simulink model "coord_test"  (R2013a)
settings: Solver=ode45  StartTime=0.0  StopTime=10.0  RelTol=1e-3
libraries: QuaternionLib x3
settings Model: Creator=EwingKang  LastModifiedBy=EwingKang

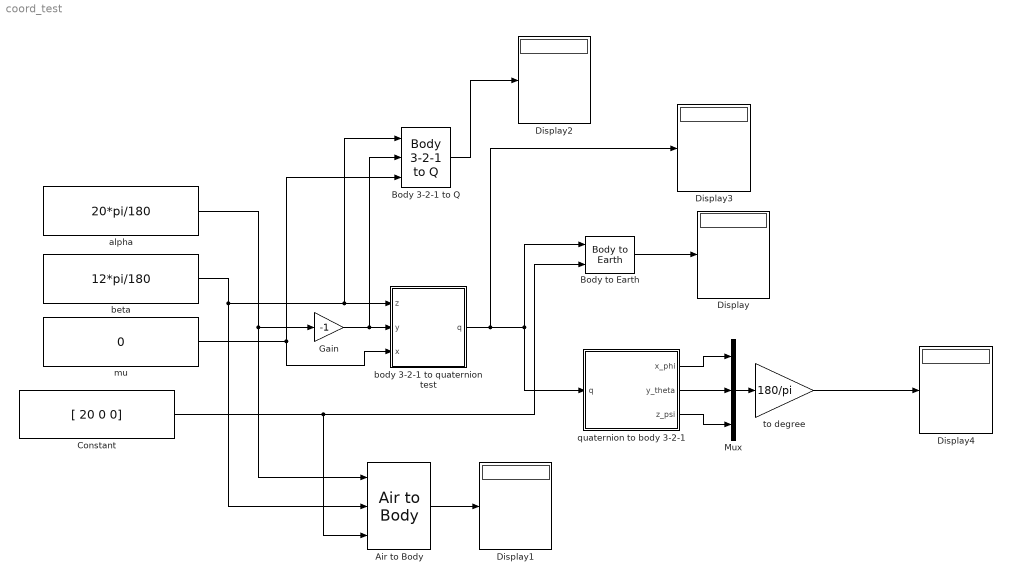
== system coord_test ==
  " quaternion to body 3-2-1" : MATLAB Function  TreatAsAtomicUnit=on
  Air to Body : QuaternionLib/Air to Body
  Body 3-2-1 to Q : QuaternionLib/Body 3-2-1 to Q
  Body to Earth : QuaternionLib/Body to Earth
  Constant : Constant  Value=[ 20 0 0]
  Display{,1..4} (5 alike) : Display
  Gain : Gain  Gain=-1
  Mux : Mux  Inputs=3
  alpha : Constant  Value=20*pi/180
  beta : Constant  Value=12*pi/180
  body 3-2-1 to quaternion test : MATLAB Function  TreatAsAtomicUnit=on
  mu : Constant  Value=0
  to degree : Gain  Gain=180/pi
  wires:
  body 3-2-1 to quaternion test/1(q) -> Display3/1, Body to Earth/1, " quaternion to body 3-2-1"/1(q)
  Constant/1 -> Air to Body/3, Body to Earth/2
  Body to Earth/1 -> Display/1
  Air to Body/1 -> Display1/1
  alpha/1 -> Air to Body/1, Gain/1
  beta/1 -> Body 3-2-1 to Q/1, body 3-2-1 to quaternion test/1(z), Air to Body/2
  mu/1 -> Body 3-2-1 to Q/3, body 3-2-1 to quaternion test/3(x)
  Gain/1 -> Body 3-2-1 to Q/2, body 3-2-1 to quaternion test/2(y)
  Body 3-2-1 to Q/1 -> Display2/1
  " quaternion to body 3-2-1"/2(y_theta) -> Mux/2
  " quaternion to body 3-2-1"/1(x_phi) -> Mux/1
  " quaternion to body 3-2-1"/3(z_psi) -> Mux/3
  Mux/1 -> to degree/1
  to degree/1 -> Display4/1

== matlab function coord_test/ quaternion to body 3-2-1 ==
  data: q input; x_phi output; y_theta output; z_psi output
function [x_phi, y_theta, z_psi] = test2(q)

q0 = q(1);
q1 = q(2);
q2 = q(3);
q3 = q(4);

x_phi = atan(  2*( q0*q1 + q2*q3 ) / ( 1 - 2*(q1^2 + q2^2 ) )  );
y_theta = asin(  2*(q0*q2-q3*q1)  );
z_psi = atan(  2*( q0*q3 + q1*q2 ) / ( 1 - 2*(q2^2 + q3^2 ) )  );
end

== matlab function coord_test/body 3-2-1 to quaternion test ==
  data: z input; q output; y input; x input
function q = test(z, y, x)
q0 = sin(x/2)*sin(y/2)*sin(z/2) + cos(x/2)*cos(y/2)*cos(z/2);         % cos(theta/2)
q1 = -cos(x/2)*sin(y/2)*sin(z/2) + sin(x/2)*cos(y/2)*cos(z/2);         % x sin(theta/2)
q2 = sin(x/2)*cos(y/2)*sin(z/2) + cos(x/2)*sin(y/2)*cos(z/2);        % y sin(theta/2)
q3 = -sin(x/2)*sin(y/2)*cos(z/2) + cos(x/2)*cos(y/2)*sin(z/2);        % z sin(theta/2)
q = zeros(1,4);
q(1) = q0;
q(2) = q1;
q(3) = q2;
q(4) = q3;
end
